simulink model "lab8"  (R2019a)
settings: Solver=ode23tb  StartTime=0.0  StopTime=10.0  RelTol=1e-5
settings Model: Creator=sumli  LastModifiedBy=sumli

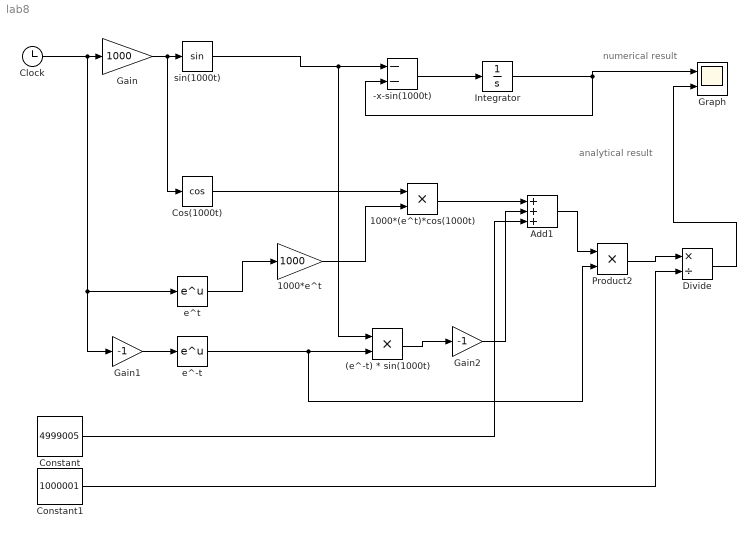
== system lab8 ==
  note: analytical result
  note: numerical result
  (e^-t) * sin(1000t) : Product
  -x-sin(1000t) : Sum  Inputs=--
  1000*(e^t)*cos(1000t) : Product
  1000*e^t : Gain  Gain=1000
  Add1 : Sum  Inputs=+++
  Clock : Clock
  Constant : Constant  Value=4999005
  Constant1 : Constant  Value=1000001
  Cos(1000t) : Trigonometry  Operator=cos
  Divide : Product  Inputs=*/
  Gain : Gain  Gain=1000
  Gain1 : Gain  Gain=-1
  Gain2 : Gain  Gain=-1
  Graph : Scope  NumInputPorts=2
  Integrator : Integrator  InitialCondition=5
  Product2 : Product
  e^-t : Math  SaturateOnIntegerOverflow=on
  e^t : Math  SaturateOnIntegerOverflow=on
  sin(1000t) : Trigonometry
  wires:
  Clock/1 -> Gain1/1, e^t/1, Gain/1
  Gain/1 -> Cos(1000t)/1, sin(1000t)/1
  Gain1/1 -> e^-t/1
  sin(1000t)/1 -> (e^-t) * sin(1000t)/1, -x-sin(1000t)/1
  Cos(1000t)/1 -> 1000*(e^t)*cos(1000t)/1
  e^t/1 -> 1000*e^t/1
  1000*e^t/1 -> 1000*(e^t)*cos(1000t)/2
  e^-t/1 -> (e^-t) * sin(1000t)/2, Product2/2
  -x-sin(1000t)/1 -> Integrator/1
  (e^-t) * sin(1000t)/1 -> Gain2/1
  1000*(e^t)*cos(1000t)/1 -> Add1/1
  Gain2/1 -> Add1/2
  Constant/1 -> Add1/3
  Integrator/1 -> Graph/1, -x-sin(1000t)/2
  Add1/1 -> Product2/1
  Product2/1 -> Divide/1
  Constant1/1 -> Divide/2
  Divide/1 -> Graph/2
